simulink library "mblibv1"  (Simulink 6.0)
settings: Solver=ode45  StartTime=0.0  StopTime=10.0  RelTol=1e-3
undefined symbols (not defined in the file or in its folder): gcbh, mech_support
libraries: mblibv1 x10, simulink x5
(part 1 of 2)
settings Model: Creator=batserve  LastModifiedBy=batserve  ExtModeAutoUpdateStatusClock=off
settings Model: ForwardingTableString=|
  | ||__slOldName__||mblibv1/Bodies/Mechanical
  | Environment||__slNewName__||mblibv1/Bodies/Machine
  | Environment||__slOldName__||mblibv1/Utilities/Convert from Pose to
  | Virtual Reality Toolbox||__slNewName__||mblibv1/Utilities/Convert from Rotation Matrix to
  | Virtual Reality Toolbox

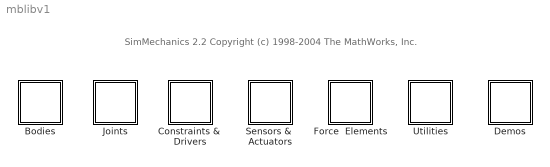
== system mblibv1 ==
  note: SimMechanics 2.2
      | Copyright (c) 1998-2004 The MathWorks, Inc.
  Bodies : Subsystem
      mask Display: image(mech_getIcon('b_lib.bmp', 'Mechanical'))
  Constraints &  Drivers : Subsystem
      mask Display: image(mech_iconLoad('private/constr_lib.bmp'))
  Demos : Subsystem
      settings: OpenFcn=demo('simulink','SimMechanics')
      mask Display: image(mech_getIcon('demo_lib.bmp', 'Mechanical'))
  Force  Elements : Subsystem
      mask Display: image(mech_getIcon('forceelements_lib.bmp', 'Mechanical'))
  Joints : Subsystem
      mask Display: image(mech_getIcon('joint_lib.bmp', 'Mechanical'))
  Sensors &  Actuators : Subsystem
      mask Display: image(mech_getIcon('s_a_lib.bmp', 'Mechanical'))
  Utilities : Subsystem
      mask Display: image(mech_getIcon('conn_lib.bmp', 'Mechanical'))

== system mblibv1/Bodies ==
  Body : PMComponent  LoadFcn=mech_support('LoadFcn',gcbh);  StartFcn=mech_support('StartFcn',gcbh);  StopFcn=mech_support('StopFcn',gcbh);  PhysicalDomain=mechanical  SubClassName=Unknown  LeftPortType=workingframe  RightPortType=workingframe  LConnTagsString=CS1  RConnTagsString=CS2  mask(msb){ClassName=Body, DialogClass=MechanicalBodyBlock, Mass=1, MassUnits=kg, InertiaUnits=kg*m^2, Inertia=eye(3), Shape=Cylinder, ShapeDims=[1 1], ShapeUnits=m, ShapeUse=false, Density=1, DensityUnits=kg/m^3, DensityUse=false, CG=None$CG$[0 0 0]$INERTIAL$INERTIAL$m$[0 0 0]$Euler X-Y-Z$deg$INERTIAL$false, WorkingFrames=Left$CS1$[0 0 0]$CG$CG$m$[0 0 0]$Euler X-Y-Z$deg$INERTIAL$true#Right$CS2$[0 0 0]$CG$CG$m$[0 0 0]$Euler X-Y-Z$deg$INERTIAL$true}
      mask prompts: Mass "MASS_VALUE"; MassUnits "MASS_UNITS"; InertiaUnits "INERTIA_UNITS"; Inertia "INERTIA_VALUE"; Shape "BASE_GEOMETRY"; ShapeDims "GEOMETRY_DIMS"; ShapeUnits "GEOMETRY_UNITS"; ShapeUse "GEOMETRY_USE"; Density "DENSITY_VALUE"; DensityUnits "DENSITY_UNITS"; DensityUse "DENSITY_USE"; CG "CG_FRAME"; WorkingFrames "WORKING_FRAMES"
      mask help: Represents a user-defined rigid body. Body defined by mass m, inertia tensor I, and coordinate origins and axes for center of gravity (CG) and other user-specified Body coordinate systems. This dialog sets Body initial position and orientation, unless Body and/or connected Joints are actuated separately.
      mask init:
      | mech_setIcon private/body.bmp
      settings: CopyFcn=mech_support('CopyFcn',gcbh);  DeleteFcn=mech_support('deleteFcn',gcbh);  UndoDeleteFcn=mech_support('undoDeleteFcn',gcbh);  ModelCloseFcn=mech_support('modelCloseFcn',gcbh);  PreSaveFcn=mech_support('PreSaveFcn');  PostSaveFcn=mech_support('PostSaveFcn');  NameChangeFcn=mech_support('nameChangeFcn',gcbh);  OpenFcn=mech_support('openFcn',gcbh);  CloseFcn=mech_support('CloseFcn',gcbh);
      mask Help: web(mech_help('body'))
      mask Display: image(mech_iconLoad('private/body.bmp'),'center');port_label('LConn',1,'CS1');port_label('RConn',1,'CS2');
  Ground : Subsystem  LoadFcn=mech_support('LoadFcn',gcbh);  StartFcn=mech_support('StartFcn',gcbh);  StopFcn=mech_support('StopFcn',gcbh);  Opaque=on  mask(msb){LeftPortType=env, RightPortType=workingframe, PhysicalDomain=Mechanical, DialogClass=GroundBlock, ClassName=Ground, CoordPosition=[0 0 0], CoordPositionUnits=m, StateVectorMgrId=-1, MachineId=[0 0], ShowEnvPort=off}
      mask help: Grounds one side of a Joint to a fixed location in the World coordinate system.
      mask init:
      | mech_initGround('ground', gcbh, MachineId);
      settings: CopyFcn=mech_support('CopyFcn',gcbh);  DeleteFcn=mech_support('deleteFcn',gcbh);  UndoDeleteFcn=mech_support('undoDeleteFcn',gcbh);  ModelCloseFcn=mech_support('modelCloseFcn',gcbh);  PreSaveFcn=mech_support('PreSaveFcn', gcbh);  PostSaveFcn=mech_support('PostSaveFcn',gcbh);  NameChangeFcn=mech_support('nameChangeFcn',gcbh);  OpenFcn=mech_support('openFcn',gcbh);  CloseFcn=mech_support('CloseFcn',gcbh);
      mask Help: web(mech_help('ground'))
      mask StyleString: edit,edit,edit,edit,edit,edit,popup(km|m|cm|mm|mi|ft|in),edit,edit,checkbox
      mask Display: image(mech_getIcon('ground.bmp', 'Mechanical'),'center','on');
  Machine Environment : Subsystem  Tag=Factory ground  DialogController=MECH.DialogSource  Opaque=on  mask(Mechanical){PortType=env, PhysicalDomain=Mechanical, ClassName=Environment, DialogTemplateClass=MECH.MachineEnvironment, SyncWhenCopied=on, Gravity=[0 -9.81 0], GravityUnits=m/s^2, GravityAsSignal=off, Dimensionality=Auto-detect, AnalysisType=Forward dynamics, LinearAssemblyTolerance=0.001, LinearAssemblyToleranceUnits=m, AngularAssemblyTolerance=0.001, AngularAssemblyToleranceUnits=rad, ConstraintSolverType=Stabilizing, ConstraintRelTolerance=0.0001, ConstraintAbsTolerance=0.0001, UseRobustSingularityHandling=off, StatePerturbationType=Adaptive, PerturbationSize=0.001, VisualizeMachine=on}
      mask help: Defines the mechanical simulation environment for the machine to which the block is connected: gravity, dimensionality, analysis mode, constraint solver type, tolerances, linearization, and visualization.
      mask init:
      | mech_environment_block('MaskInitialization', gcbh);
      settings: CopyFcn=mech_environment_block('CopyFcn', gcbh);
      mask Help: web(mech_help('machineenvironment'))
      mask StyleString: edit,edit,edit,edit,edit,edit,popup(km/s^2|m/s^2|cm/s^2|mm/s^2|mi/s^2|ft/s^2|in/s^2),checkbox,popup(2D Only|3D Only|Auto-detect),popup(Forward dynamics|Inverse dynamics|Kinematics|Trimming),edit,popup(km|m|cm|mm|mi|ft|in),edit,popup(deg|rad),popup(Stabilizing|Tolerancing|Machine precision),edit,edit,checkbox,popup(Adaptive|Fixed),edit,checkbox
      mask Display: disp('Env')

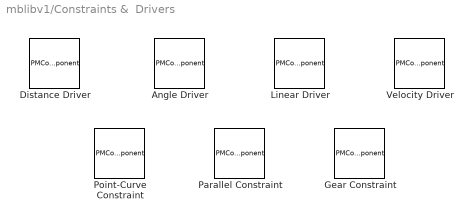
== system mblibv1/Constraints &  Drivers ==
  Angle Driver : PMComponent  LoadFcn=mech_support('LoadFcn',gcbh);  StartFcn=mech_support('StartFcn',gcbh);  StopFcn=mech_support('StopFcn',gcbh);  PhysicalDomain=mechanical  SubClassName=Unknown  LeftPortType=blob  RightPortType=blob  LConnTagsString=__newl0  RConnTagsString=__newr0  mask(AngleDriverConstraint){ClassName=AngleDriver, DialogClass=AngleDriverConstraint, NumSAPorts=0, LeftCsys=WORLD, RightCsys=WORLD, LeftAxis=[1 0 0], RightAxis=[1 0 0]}
      mask help: Drives the angle between base (B) and follower (F) Body axis vectors with a specified Driver Actuator signal, which is added to the initial condition. An unactuated Driver holds the angle in its initial state. Fixed axes define body axis vectors in base and follower coordinate systems. Sensor and actuator ports can be added. Base-follower sequence determines sign of forward motion.
      settings: CopyFcn=mech_support('CopyFcn',gcbh);  DeleteFcn=mech_support('deleteFcn',gcbh);  UndoDeleteFcn=mech_support('undoDeleteFcn',gcbh);  ModelCloseFcn=mech_support('modelCloseFcn',gcbh);  NameChangeFcn=mech_support('nameChangeFcn',gcbh);  OpenFcn=mech_support('openFcn',gcbh);  CloseFcn=mech_support('CloseFcn',gcbh);
      mask Help: web(mech_help('angledriver'))
      mask Display: image(mech_getIcon('ang_drvr.bmp', 'Mechanical'),'center');color('magenta'); port_label('LConn',1,'B'); port_label('RConn',1,'F')
  Distance Driver : PMComponent  LoadFcn=mech_support('LoadFcn',gcbh);  StartFcn=mech_support('StartFcn',gcbh);  StopFcn=mech_support('StopFcn',gcbh);  PhysicalDomain=mechanical  SubClassName=Unknown  LeftPortType=blob  RightPortType=blob  LConnTagsString=__newl0  RConnTagsString=__newr0  mask(DistanceDriverConstraint){ClassName=DistanceDriver, DialogClass=DistanceDriverConstraint, NumSAPorts=0}
      mask help: Drives the distance between origins of the base (B) and follower (F) Body coordinate systems with a specified Driver Actuator signal, which is added to the initial condition. An unactuated Driver holds the distance in its initial state. Distance must remain non-negative at all times. Sensor and actuator ports can be added.
      settings: CopyFcn=mech_support('CopyFcn',gcbh);  DeleteFcn=mech_support('deleteFcn',gcbh);  UndoDeleteFcn=mech_support('undoDeleteFcn',gcbh);  ModelCloseFcn=mech_support('modelCloseFcn',gcbh);  NameChangeFcn=mech_support('nameChangeFcn',gcbh);  OpenFcn=mech_support('openFcn',gcbh);  CloseFcn=mech_support('CloseFcn',gcbh);
      mask Help: web(mech_help('distancedriver'))
      mask Display: image(mech_getIcon('dist_drvr.bmp', 'Mechanical'),'center');color('magenta'); port_label('LConn',1,'B'); port_label('RConn',1,'F')
  Gear Constraint : PMComponent  LoadFcn=mech_support('LoadFcn',gcbh);  StartFcn=mech_support('StartFcn',gcbh);  StopFcn=mech_support('StopFcn',gcbh);  PhysicalDomain=mechanical  SubClassName=Unknown  LeftPortType=blob  RightPortType=blob  LConnTagsString=__newl0  RConnTagsString=__newr0  mask(GearConstraint){ClassName=GearConstraint, DialogClass=GearConstraint, NumSAPorts=0, BaseRadius=1, BaseRadiusUnits=m, FollowerRadius=1, FollowerRadiusUnits=m}
      mask help: Constrains the base (B) and follower (F) Bodies to corotate as meshed gears with pitch circles. The base and follower Bodies must be attached to a third, carrier Body by Revolute or Cylindrical Joints. These joints define the gear rotational axes. Sensor ports can be added. Base-follower sequence determines sign of forward motion.
      settings: CopyFcn=mech_support('CopyFcn',gcbh);  DeleteFcn=mech_support('deleteFcn',gcbh);  UndoDeleteFcn=mech_support('undoDeleteFcn',gcbh);  ModelCloseFcn=mech_support('modelCloseFcn',gcbh);  NameChangeFcn=mech_support('nameChangeFcn',gcbh);  OpenFcn=mech_support('openFcn',gcbh);  CloseFcn=mech_support('CloseFcn',gcbh);
      mask Help: web(mech_help('gearconstraint'))
      mask Display: image(mech_getIcon('gear.bmp', 'Mechanical'),'center');color('magenta'); port_label('LConn',1,'B'); port_label('RConn',1,'F')
  Linear Driver : PMComponent  LoadFcn=mech_support('LoadFcn',gcbh);  StartFcn=mech_support('StartFcn',gcbh);  StopFcn=mech_support('StopFcn',gcbh);  PhysicalDomain=mechanical  SubClassName=Unknown  LeftPortType=blob  RightPortType=blob  LConnTagsString=__newl0  RConnTagsString=__newr0  mask(LinearDriverConstraint){ClassName=LinearDriver, DialogClass=LinearDriverConstraint, NumSAPorts=0, GlobalCoordinate=X}
      mask help: Drives one component [X, Y, or Z] of the relative vector between the origins of the base (B) and follower (F) Body coordinate systems with a Driver Actuator signal, which is added to the initial condition. An unactuated Driver holds the component in its initial state. Vector component measured with respect to the World coordinate system. Follower is the head and base is the tail of relative vector. Sensor and actuator ports can be added. Base-follower sequence determines sign of forward motion, including relative vector component signs.
      settings: CopyFcn=mech_support('CopyFcn',gcbh);  DeleteFcn=mech_support('deleteFcn',gcbh);  UndoDeleteFcn=mech_support('undoDeleteFcn',gcbh);  ModelCloseFcn=mech_support('modelCloseFcn',gcbh);  NameChangeFcn=mech_support('nameChangeFcn',gcbh);  OpenFcn=mech_support('openFcn',gcbh);  CloseFcn=mech_support('CloseFcn',gcbh);
      mask Help: web(mech_help('lineardriver'))
      mask Display: image(mech_getIcon('lin_drvr.bmp', 'Mechanical'),'center');color('magenta'); port_label('LConn',1,'B'); port_label('RConn',1,'F')
  Parallel Constraint : PMComponent  LoadFcn=mech_support('LoadFcn',gcbh);  StartFcn=mech_support('StartFcn',gcbh);  StopFcn=mech_support('StopFcn',gcbh);  PhysicalDomain=mechanical  SubClassName=Unknown  LeftPortType=blob  RightPortType=blob  LConnTagsString=__newl0  RConnTagsString=__newr0  mask(ParallelConstraint){ClassName=ParallelConstraint, DialogClass=ParallelConstraint, NumSAPorts=0, Csys=WORLD, Axis=[1 0 0]}
      mask help: Constrains one Body axis vector defined on both base (B) and follower (F) Bodies to remain parallel. Parallel constraint axis defines initial direction of both Body axis vectors in base and follower Body coordinate systems. Sensor ports can be added. Base-follower sequence determines sign of forward motion.
      settings: CopyFcn=mech_support('CopyFcn',gcbh);  DeleteFcn=mech_support('deleteFcn',gcbh);  UndoDeleteFcn=mech_support('undoDeleteFcn',gcbh);  ModelCloseFcn=mech_support('modelCloseFcn',gcbh);  NameChangeFcn=mech_support('nameChangeFcn',gcbh);  OpenFcn=mech_support('openFcn',gcbh);  CloseFcn=mech_support('CloseFcn',gcbh);
      mask Help: web(mech_help('parallelconstraint'))
      mask Display: image(mech_getIcon('parallel.bmp', 'Mechanical'),'center');color('magenta'); port_label('LConn',1,'B'); port_label('RConn',1,'F')
  Point-Curve Constraint : PMComponent  LoadFcn=mech_support('LoadFcn',gcbh);  StartFcn=mech_support('StartFcn',gcbh);  StopFcn=mech_support('StopFcn',gcbh);  PhysicalDomain=mechanical  SubClassName=Unknown  LeftPortType=blob  RightPortType=blob  LConnTagsString=__newl0  RConnTagsString=__newr0  mask(PointCurveConstraint){ClassName=PointCurve, DialogClass=PointCurveConstraint, Units=m, Xbreaks=[  ], Ybreaks=[  ], Zbreaks=[  ], EndConditions=natural, CanExtrapolate=off, NumSAPorts=0}
      mask help: Constrains the Body coordinate system origin on Body (B) to move along a curve defined in the Body coordinate system on Body (F). The curve is defined as a spline with breakpoints. Sensor ports can be added. Base-follower sequence determines sign of forward motion.
      settings: CopyFcn=mech_support('CopyFcn',gcbh);  DeleteFcn=mech_support('deleteFcn',gcbh);  UndoDeleteFcn=mech_support('undoDeleteFcn',gcbh);  ModelCloseFcn=mech_support('modelCloseFcn',gcbh);  NameChangeFcn=mech_support('nameChangeFcn',gcbh);  OpenFcn=mech_support('openFcn',gcbh);  CloseFcn=mech_support('CloseFcn',gcbh);
      mask Help: web(mech_help('pointcurveconstraint'))
      mask Display: color('magenta');image(mech_getIcon('pt_curve.bmp','Mechanical'),'center');port_label('LConn',1,'B'); port_label('RConn',1,'F')
  Velocity Driver : PMComponent  LoadFcn=mech_support('LoadFcn',gcbh);  StartFcn=mech_support('StartFcn',gcbh);  StopFcn=mech_support('StopFcn',gcbh);  PhysicalDomain=mechanical  SubClassName=Unknown  LeftPortType=blob  RightPortType=blob  LConnTagsString=__newl0  RConnTagsString=__newr0  mask(ConstantVelocityConstraint){ClassName=ConstantVelocity, DialogClass=ConstantVelocityConstraint, NumSAPorts=0, Unit_V=m/s, Unit_Omega=deg/s, Coef_V_Base=[1 0 0], Csys_V_Base=WORLD, Coef_Omega_Base=[1 0 0], Csys_Omega_Base=WORLD, Coef_V_Follower=[1 0 0], Csys_V_Follower=WORLD, Coef_Omega_Follower=[1 0 0], Csys_Omega_Follower=WORLD}
      mask help: Drives a linear combination of projected linear and angular velocities of the base (B) and follower (F) Bodies with a specified Driver Actuator signal, which is added to the initial condition. An unactuated Driver holds the linear combination in its initial state. Sensor and actuator ports can be added. Base-follower sequence determines sign of forward motion.
      settings: CopyFcn=mech_support('CopyFcn',gcbh);  DeleteFcn=mech_support('deleteFcn',gcbh);  UndoDeleteFcn=mech_support('undoDeleteFcn',gcbh);  ModelCloseFcn=mech_support('modelCloseFcn',gcbh);  NameChangeFcn=mech_support('nameChangeFcn',gcbh);  OpenFcn=mech_support('openFcn',gcbh);  CloseFcn=mech_support('CloseFcn',gcbh);
      mask Help: web(mech_help('velocitydriver'))
      mask Display: image(mech_getIcon('con_vel.bmp', 'Mechanical'),'center');color('magenta'); port_label('LConn',1,'B'); port_label('RConn',1,'F')

== system mblibv1/Demos ==

== system mblibv1/Force  Elements ==
  Body Spring & Damper : Subsystem  LoadFcn=mech_support('LoadFcn',gcbh);  StartFcn=mech_support('StartFcn',gcbh);  StopFcn=mech_support('StopFcn',gcbh);  mask(msb){ClassName=BodyForceElement, DialogClass=BodySpringDamper, Spring_k=0, Damper_b=0, Offset_x0=0, PositionUnits=m, VelocityUnits=m/s, ForceUnits=N}
      mask help: Models a damped linear oscillator between two Bodies, equivalent to a translational spring and damper. The force F between the bodies is projected along the axis connecting the Body coordinate systems and is a function of the relative displacement r and velocity v of these Body coordinate systems, given by F = -k*(r-r0) - b*v. The parameters r0, k, and b represent the spring's natural length, the spring constant, and the damper constant, respectively.
      mask init:
      | mech_support('MaskInit', gcbh);
      settings: CopyFcn=mech_support('CopyFcn',gcbh);  DeleteFcn=mech_support('deleteFcn',gcbh);  UndoDeleteFcn=mech_support('undoDeleteFcn',gcbh);  ModelCloseFcn=mech_support('modelCloseFcn',gcbh);  NameChangeFcn=mech_support('nameChangeFcn',gcbh);  OpenFcn=mech_support('openFcn',gcbh);  CloseFcn=mech_support('CloseFcn',gcbh);
      mask Help: web(mech_help('bodyspringdamper'))
      mask Display: image(mech_getIcon('body_springdamper.bmp', 'Mechanical'),'center')
  Joint Spring & Damper : Subsystem  LoadFcn=mech_support('LoadFcn',gcbh);  StartFcn=mech_support('StartFcn',gcbh);  StopFcn=mech_support('StopFcn',gcbh);  mask(msb){ClassName=JointSpringDamper, DialogClass=JointSpringDamper, JFEParameters=P1$false$0$0$0$m$m/s$N$rad$rad/s$N-m#P2$false$0$0$0$m$m/s$N$rad$rad/s$N-m#P3$false$0$0$0$m$m/s$N$rad$rad/s$N-m#R1$false$0$0$0$m$m/s$N$rad$rad/s$N-m#R2$false$0$0$0$m$m/s$N$rad$rad/s$N-m#R3$false$0$0$0$m$m/s$N$rad$rad/s$N-m#S$false$0$0$0$m$m/s$N$rad$rad/s$N-m}
      mask help: Models a damped linear oscillator in a Joint connecting two Bodies, equivalent to a translational spring and damper on prismatic primitives and a torsional spring and damper on revolute primitives. The force or torque F between the bodies is a function of the relative linear or angular displacement x and the linear or angular velocity v of the bodies, given by F = -k*(x-x0) - b*v. The parameters x0, k, and b represent the spring offset, spring constant, and damper constant, respectively. Each prismatic and revolute primitive has a separate spring.
      mask init:
      | mech_support('MaskInit', gcbh);
      settings: CopyFcn=mech_support('CopyFcn',gcbh);  DeleteFcn=mech_support('deleteFcn',gcbh);  UndoDeleteFcn=mech_support('undoDeleteFcn',gcbh);  ModelCloseFcn=mech_support('modelCloseFcn',gcbh);  PreSaveFcn=mech_support('PreSaveFcn');  PostSaveFcn=mech_support('PostSaveFcn');  NameChangeFcn=mech_support('nameChangeFcn',gcbh);  OpenFcn=mech_support('openFcn',gcbh);  CloseFcn=mech_support('CloseFcn',gcbh);
      mask Help: web(mech_help('jointspringdamper'))
      mask Display: image(mech_getIcon('joint_springdamper.bmp', 'Mechanical'),'center')

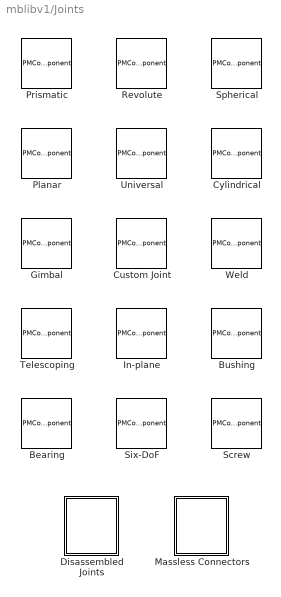
== system mblibv1/Joints ==
  Bearing : PMComponent  LoadFcn=mech_support('LoadFcn',gcbh);  StartFcn=mech_support('StartFcn',gcbh);  StopFcn=mech_support('StopFcn',gcbh);  PhysicalDomain=mechanical  SubClassName=Unknown  LeftPortType=blob  RightPortType=blob  LConnTagsString=__newl0  RConnTagsString=__newr0  mask(msb){NumSAPorts=0, CutJoint=off, MarkAsCut=off, Primitives=revolute_revolute_revolute_prismatic, PrimitiveProps=R1$INERTIAL$[1 0 0]$revolute#R2$INERTIAL$[0 1 0]$revolute#R3$INERTIAL$[0 0 1]$revolute#P1$INERTIAL$[0 0 1]$prismatic, ClassName=BearingJoint, DialogClass=JointBlock}
      mask help: Represents three rotational and one translational degrees of freedom. The follower (F) rotates around three primitive revolute axes (R1, R2, R3) and translates along one primitive prismatic axis P1 with respect to the base (B) Body. Axis P1 must be parallel to axis R3. R1 attached to base. P1 attached to follower. Listed order of primitives is order of motion during simulation. Sensor and actuator ports can be added. Base-follower sequence and axes directions determine sign of forward motion. This joint becomes singular if two revolutes align.
      settings: CopyFcn=mech_support('CopyFcn',gcbh);  DeleteFcn=mech_support('deleteFcn',gcbh);  UndoDeleteFcn=mech_support('undoDeleteFcn',gcbh);  ModelCloseFcn=mech_support('modelCloseFcn',gcbh);  PreSaveFcn=mech_support('PreSaveFcn');  PostSaveFcn=mech_support('PostSaveFcn');  NameChangeFcn=mech_support('nameChangeFcn',gcbh);  OpenFcn=mech_support('openFcn',gcbh);  CloseFcn=mech_support('CloseFcn',gcbh);
      mask Help: web(mech_help('bearing'))
      mask Display: image(mech_getIcon('bearing.bmp', 'Mechanical'),'center');color('red');text(mech_cutAffordance('offset', gcbh) - 2, 0, mech_cutAffordance('text', gcbh),'HorizontalAlignment', 'right','VerticalAlignment', 'bottom');color('magenta');port_label('LConn', 1, 'B');port_label('RConn', 1, 'F');
  Bushing : PMComponent  LoadFcn=mech_support('LoadFcn',gcbh);  StartFcn=mech_support('StartFcn',gcbh);  StopFcn=mech_support('StopFcn',gcbh);  PhysicalDomain=mechanical  SubClassName=Unknown  LeftPortType=blob  RightPortType=blob  LConnTagsString=__newl0  RConnTagsString=__newr0  mask(msb){NumSAPorts=0, CutJoint=off, MarkAsCut=off, Primitives=prismatic_prismatic_prismatic_revolute_revolute_revolute, PrimitiveProps=P1$INERTIAL$[1 0 0]$prismatic#P2$INERTIAL$[0 1 0]$prismatic#P3$INERTIAL$[0 0 1]$prismatic#R1$INERTIAL$[1 0 0]$revolute#R2$INERTIAL$[0 1 0]$revolute#R3$INERTIAL$[0 0 1]$revolute, ClassName=Joint, DialogClass=JointBlock}
      mask help: Represents three rotational and three translational degrees of freedom. The follower (F) translates along three primitive prismatic axes (P1, P2, P3) and rotates around three primitive revolute axes (R1, R2, R3) relative to the base (B) Body. P1 attached to base. R3 attached to follower. Listed order of primitives is order of motion during simulation. Sensor and actuator ports can be added. Base-follower sequence and axes directions determine sign of forward motion. This joint becomes singular if two prismatics or two revolutes align.
      settings: CopyFcn=mech_support('CopyFcn',gcbh);  DeleteFcn=mech_support('deleteFcn',gcbh);  UndoDeleteFcn=mech_support('undoDeleteFcn',gcbh);  ModelCloseFcn=mech_support('modelCloseFcn',gcbh);  PreSaveFcn=mech_support('PreSaveFcn');  PostSaveFcn=mech_support('PostSaveFcn');  NameChangeFcn=mech_support('nameChangeFcn',gcbh);  OpenFcn=mech_support('openFcn',gcbh);  CloseFcn=mech_support('CloseFcn',gcbh);
      mask Help: web(mech_help('bushing'))
      mask Display: image(mech_getIcon('bushing.bmp', 'Mechanical'),'center');color('red');text(mech_cutAffordance('offset', gcbh) - 2, 0, mech_cutAffordance('text', gcbh),'HorizontalAlignment', 'right','VerticalAlignment', 'bottom');color('magenta');port_label('LConn', 1, 'B');port_label('RConn', 1, 'F');
  Custom Joint : PMComponent  LoadFcn=mech_support('LoadFcn',gcbh);  StartFcn=mech_support('StartFcn',gcbh);  StopFcn=mech_support('StopFcn',gcbh);  PhysicalDomain=mechanical  SubClassName=custom_joint  LeftPortType=blob  RightPortType=blob  LConnTagsString=__newl0  RConnTagsString=__newr0  mask(msb){NumSAPorts=0, CutJoint=off, MarkAsCut=off, Primitives=revolute, PrimitiveProps=R1$INERTIAL$[0 0 1]$revolute, ClassName=Joint, DialogClass=JointBlock}
      mask help: Represents general user-defined joint with multiple degrees of freedom. Connects two Bodies with combination of prismatic, revolute, and/or spherical primitives. This Joint limited to maximum of six DoFs: up to three rotational DoFs and up to three translational DoFs. First primitive attached to base (B). Last primitive attached to follower (F). Listed order of primitives is order of motion during simulation. Sensor and actuator ports can be added. Spherical primitive cannot be actuated. Base-follower sequence and axes directions determine sign of forward motion.This joint becomes singular if two prismatics or two revolutes align.
      settings: CopyFcn=mech_support('CopyFcn',gcbh);  DeleteFcn=mech_support('deleteFcn',gcbh);  UndoDeleteFcn=mech_support('undoDeleteFcn',gcbh);  ModelCloseFcn=mech_support('modelCloseFcn',gcbh);  PreSaveFcn=mech_support('PreSaveFcn');  PostSaveFcn=mech_support('PostSaveFcn');  NameChangeFcn=mech_support('nameChangeFcn',gcbh);  OpenFcn=mech_support('openFcn',gcbh);  CloseFcn=mech_support('CloseFcn',gcbh);
      mask Help: web(mech_help('customjoint'))
      mask Display: image(mech_getIcon('comp_joint.bmp', 'Mechanical'),'center');color('red');text(mech_cutAffordance('offset', gcbh) - 2, 0, mech_cutAffordance('text', gcbh),'HorizontalAlignment', 'right','VerticalAlignment', 'bottom');color('magenta');port_label('LConn', 1, 'B');port_label('RConn', 1, 'F');
  Cylindrical : PMComponent  LoadFcn=mech_support('LoadFcn',gcbh);  StartFcn=mech_support('StartFcn',gcbh);  StopFcn=mech_support('StopFcn',gcbh);  PhysicalDomain=mechanical  SubClassName=Unknown  LeftPortType=blob  RightPortType=blob  LConnTagsString=__newl0  RConnTagsString=__newr0  mask(msb){NumSAPorts=0, CutJoint=off, MarkAsCut=off, Primitives=prismatic_revolute, PrimitiveProps=P1$INERTIAL$[1 0 0]$prismatic#R1$INERTIAL$[1 0 0]$revolute, ClassName=CylindricalJoint, DialogClass=JointBlock}
      mask help: Represents one translational and one rotational degrees of freedom. Restricts the follower (F) to move relative to the base (B) Body along and around a common axis P1-R1. Primitive axes P1 and R1 must be aligned. P1 attached to base. R1 attached to follower. Listed order of primitives is order of motion during simulation. Sensor and actuator ports can be added. Base-follower sequence and axis direction determine sign of forward motion.
      settings: CopyFcn=mech_support('CopyFcn',gcbh);  DeleteFcn=mech_support('deleteFcn',gcbh);  UndoDeleteFcn=mech_support('undoDeleteFcn',gcbh);  ModelCloseFcn=mech_support('modelCloseFcn',gcbh);  PreSaveFcn=mech_support('PreSaveFcn');  PostSaveFcn=mech_support('PostSaveFcn');  NameChangeFcn=mech_support('nameChangeFcn',gcbh);  OpenFcn=mech_support('openFcn',gcbh);  CloseFcn=mech_support('CloseFcn',gcbh);
      mask Help: web(mech_help('cylindrical'))
      mask Display: image(mech_getIcon('cylindrical.bmp', 'Mechanical'),'center');color('red');text(mech_cutAffordance('offset', gcbh) - 2, 0, mech_cutAffordance('text', gcbh),'HorizontalAlignment', 'right','VerticalAlignment', 'bottom');color('magenta');port_label('LConn', 1, 'B');port_label('RConn', 1, 'F');
  Disassembled Joints : Subsystem
      mask Display: image(mech_getIcon('joint_lib.bmp', 'Mechanical'))
  Gimbal : PMComponent  LoadFcn=mech_support('LoadFcn',gcbh);  StartFcn=mech_support('StartFcn',gcbh);  StopFcn=mech_support('StopFcn',gcbh);  PhysicalDomain=mechanical  SubClassName=Unknown  LeftPortType=blob  RightPortType=blob  LConnTagsString=__newl0  RConnTagsString=__newr0  mask(msb){NumSAPorts=0, CutJoint=off, MarkAsCut=off, Primitives=revolute_revolute_revolute, PrimitiveProps=R1$INERTIAL$[1 0 0]$revolute#R2$INERTIAL$[0 1 0]$revolute#R3$INERTIAL$[0 0 1]$revolute, ClassName=Joint, DialogClass=JointBlock}
      mask help: Represents three rotational degrees of freedom. The follower (F) rotates with respect to the base (B) Body around three primitive revolute axes (R1, R2, R3). R1 attached to base. R3 attached to follower. Listed order of primitives is order of motion during simulation. Sensor and actuator ports can be added. Base-follower sequence and axes directions determine sign of forward motion. This joint becomes singular if two revolutes align.
      settings: CopyFcn=mech_support('CopyFcn',gcbh);  DeleteFcn=mech_support('deleteFcn',gcbh);  UndoDeleteFcn=mech_support('undoDeleteFcn',gcbh);  ModelCloseFcn=mech_support('modelCloseFcn',gcbh);  PreSaveFcn=mech_support('PreSaveFcn');  PostSaveFcn=mech_support('PostSaveFcn');  NameChangeFcn=mech_support('nameChangeFcn',gcbh);  OpenFcn=mech_support('openFcn',gcbh);  CloseFcn=mech_support('CloseFcn',gcbh);
      mask Help: web(mech_help('gimbal'))
      mask Display: image(mech_getIcon('gimbal.bmp', 'Mechanical'),'center');color('red');text(mech_cutAffordance('offset', gcbh) - 2, 0, mech_cutAffordance('text', gcbh),'HorizontalAlignment', 'right','VerticalAlignment', 'bottom');color('magenta');port_label('LConn', 1, 'B');port_label('RConn', 1, 'F');
  In-plane : PMComponent  LoadFcn=mech_support('LoadFcn',gcbh);  StartFcn=mech_support('StartFcn',gcbh);  StopFcn=mech_support('StopFcn',gcbh);  PhysicalDomain=mechanical  SubClassName=Unknown  LeftPortType=blob  RightPortType=blob  LConnTagsString=__newl0  RConnTagsString=__newr0  mask(msb){NumSAPorts=0, CutJoint=off, MarkAsCut=off, Primitives=prismatic_prismatic, PrimitiveProps=P1$INERTIAL$[1 0 0]$prismatic#P2$INERTIAL$[0 1 0]$prismatic, ClassName=InplaneJoint, DialogClass=JointBlock}
      mask help: Represents two translational degrees of freedom. Restricts the follower (F) to move relative to the base (B) Body in plane defined by span of two primitive prismatic axes (P1, P2). P1 attached to base. P2 attached to follower. Listed order of primitives is order of motion during simulation. Sensor and actuator ports can be added. Base-follower sequence and axes directions determine sign of forward motion. This joint becomes singular if both prismatics align.
      settings: CopyFcn=mech_support('CopyFcn',gcbh);  DeleteFcn=mech_support('deleteFcn',gcbh);  UndoDeleteFcn=mech_support('undoDeleteFcn',gcbh);  ModelCloseFcn=mech_support('modelCloseFcn',gcbh);  PreSaveFcn=mech_support('PreSaveFcn');  PostSaveFcn=mech_support('PostSaveFcn');  NameChangeFcn=mech_support('nameChangeFcn',gcbh);  OpenFcn=mech_support('openFcn',gcbh);  CloseFcn=mech_support('CloseFcn',gcbh);
      mask Help: web(mech_help('inplane'))
      mask Display: image(mech_getIcon('inplane.bmp', 'Mechanical'),'center');color('red');text(mech_cutAffordance('offset', gcbh) - 2, 0, mech_cutAffordance('text', gcbh),'HorizontalAlignment', 'right','VerticalAlignment', 'bottom');color('magenta');port_label('LConn', 1, 'B');port_label('RConn', 1, 'F');
  Massless Connectors : Subsystem
      mask Display: image(mech_getIcon('joint_lib.bmp', 'Mechanical'))
  Planar : PMComponent  LoadFcn=mech_support('LoadFcn',gcbh);  StartFcn=mech_support('StartFcn',gcbh);  StopFcn=mech_support('StopFcn',gcbh);  PhysicalDomain=mechanical  SubClassName=Unknown  LeftPortType=blob  RightPortType=blob  LConnTagsString=__newl0  RConnTagsString=__newr0  mask(msb){NumSAPorts=0, CutJoint=off, MarkAsCut=off, Primitives=prismatic_prismatic_revolute, PrimitiveProps=P1$INERTIAL$[1 0 0]$prismatic#P2$INERTIAL$[0 1 0]$prismatic#R1$INERTIAL$[0 0 1]$revolute, ClassName=PlanarJoint, DialogClass=JointBlock}
      mask help: Represents two translational and one rotational degrees of freedom. Restricts the follower (F) to move relative to the base (B) Body in plane defined by span of two primitive prismatic axes (P1, P2). follower can also rotate about axis R1 = P1 x P2. Axis R1 must be normal to plane. P1 attached to base. R1 attached to follower. Listed order of primitives is order of motion during simulation. Sensor and actuator ports can be added. Base-follower sequence and axes directions determine sign of forward motion. This joint becomes singular if both prismatics align.
      settings: CopyFcn=mech_support('CopyFcn',gcbh);  DeleteFcn=mech_support('deleteFcn',gcbh);  UndoDeleteFcn=mech_support('undoDeleteFcn',gcbh);  ModelCloseFcn=mech_support('modelCloseFcn',gcbh);  PreSaveFcn=mech_support('PreSaveFcn');  PostSaveFcn=mech_support('PostSaveFcn');  NameChangeFcn=mech_support('nameChangeFcn',gcbh);  OpenFcn=mech_support('openFcn',gcbh);  CloseFcn=mech_support('CloseFcn',gcbh);
      mask Help: web(mech_help('planar'))
      mask Display: image(mech_getIcon('planar.bmp', 'Mechanical'),'center');color('red');text(mech_cutAffordance('offset', gcbh) - 2, 0, mech_cutAffordance('text', gcbh),'HorizontalAlignment', 'right','VerticalAlignment', 'bottom');color('magenta');port_label('LConn', 1, 'B');port_label('RConn', 1, 'F');
  Prismatic : PMComponent  LoadFcn=mech_support('LoadFcn',gcbh);  StartFcn=mech_support('StartFcn',gcbh);  StopFcn=mech_support('StopFcn',gcbh);  PhysicalDomain=mechanical  SubClassName=Unknown  LeftPortType=blob  RightPortType=blob  LConnTagsString=__newl0  RConnTagsString=__newr0  mask(msb){NumSAPorts=0, CutJoint=off, MarkAsCut=off, Primitives=prismatic, PrimitiveProps=P1$INERTIAL$[0 0 1]$prismatic, ClassName=Joint, DialogClass=JointBlock}
      mask help: Represents one translational degree of freedom. The follower (F) body translates relative to the base (B) Body along single translational axis connecting Body coordinate origins. Sensor and actuator ports can be added. Base-follower sequence and axis direction determine sign of forward motion.
      settings: CopyFcn=mech_support('CopyFcn',gcbh);  DeleteFcn=mech_support('deleteFcn',gcbh);  UndoDeleteFcn=mech_support('undoDeleteFcn',gcbh);  ModelCloseFcn=mech_support('modelCloseFcn',gcbh);  PreSaveFcn=mech_support('PreSaveFcn');  PostSaveFcn=mech_support('PostSaveFcn');  NameChangeFcn=mech_support('nameChangeFcn',gcbh);  OpenFcn=mech_support('openFcn',gcbh);  CloseFcn=mech_support('CloseFcn',gcbh);
      mask Help: web(mech_help('prismatic'))
      mask Display: image(mech_getIcon('prismatic.bmp', 'Mechanical'),'center');color('red');text(mech_cutAffordance('offset', gcbh) - 2, 0, mech_cutAffordance('text', gcbh),'HorizontalAlignment', 'right','VerticalAlignment', 'bottom');color('magenta');port_label('LConn', 1, 'B');port_label('RConn', 1, 'F');
  Revolute : PMComponent  LoadFcn=mech_support('LoadFcn',gcbh);  StartFcn=mech_support('StartFcn',gcbh);  StopFcn=mech_support('StopFcn',gcbh);  PhysicalDomain=mechanical  SubClassName=Unknown  LeftPortType=blob  RightPortType=blob  LConnTagsString=__newl0  RConnTagsString=__newr0  mask(msb){NumSAPorts=0, CutJoint=off, MarkAsCut=off, Primitives=revolute, PrimitiveProps=R1$INERTIAL$[0 0 1]$revolute, ClassName=Joint, DialogClass=JointBlock}
      mask help: Represents one rotational degree of freedom. The follower (F) Body rotates relative to the base (B) Body about a single rotational axis going through collocated Body coordinate system origins. Sensor and actuator ports can be added. Base-follower sequence and axis direction determine sign of forward motion by the right-hand rule.
      settings: CopyFcn=mech_support('CopyFcn',gcbh);  DeleteFcn=mech_support('deleteFcn',gcbh);  UndoDeleteFcn=mech_support('undoDeleteFcn',gcbh);  ModelCloseFcn=mech_support('modelCloseFcn',gcbh);  PreSaveFcn=mech_support('PreSaveFcn');  PostSaveFcn=mech_support('PostSaveFcn');  NameChangeFcn=mech_support('nameChangeFcn',gcbh);  OpenFcn=mech_support('openFcn',gcbh);  CloseFcn=mech_support('CloseFcn',gcbh);
      mask Help: web(mech_help('revolute'))
      mask Display: image(mech_getIcon('revolute.bmp', 'Mechanical'),'center');color('red');text(mech_cutAffordance('offset', gcbh) - 2, 0, mech_cutAffordance('text', gcbh),'HorizontalAlignment', 'right','VerticalAlignment', 'bottom');color('magenta');port_label('LConn', 1, 'B');port_label('RConn', 1, 'F');
  Screw : PMComponent  LoadFcn=mech_support('LoadFcn',gcbh);  StartFcn=mech_support('StartFcn',gcbh);  StopFcn=mech_support('StopFcn',gcbh);  PhysicalDomain=mechanical  SubClassName=Unknown  LeftPortType=blob  RightPortType=blob  LConnTagsString=__newl0  RConnTagsString=__newr0  mask(msb){NumSAPorts=0, CutJoint=off, MarkAsCut=off, Primitives=revolute, PrimitiveProps=R1$INERTIAL$[1 0 0]$revolute, ClassName=ScrewJoint, DialogClass=ScrewJointBlock, Pitch=1, Units=mm}
      mask help: Represents one translational and one rotational degrees of freedom, with constraint. Restricts the follower (F) to move in helical motion along and around axis R1 relative to the base (B) Body. Translation and rotation constrained to each other by pitch. R1 attached to base and follower. Sensor and actuator ports can be added. Base-follower sequence and axis direction determine sign of forward motion.
      settings: CopyFcn=mech_support('CopyFcn',gcbh);  DeleteFcn=mech_support('deleteFcn',gcbh);  UndoDeleteFcn=mech_support('undoDeleteFcn',gcbh);  ModelCloseFcn=mech_support('modelCloseFcn',gcbh);  PreSaveFcn=mech_support('PreSaveFcn');  PostSaveFcn=mech_support('PostSaveFcn');  NameChangeFcn=mech_support('nameChangeFcn',gcbh);  OpenFcn=mech_support('openFcn',gcbh);  CloseFcn=mech_support('CloseFcn',gcbh);
      mask Help: web(mech_help('screw'))
      mask Display: image(mech_getIcon('screw.bmp', 'Mechanical'),'center');color('red');text(mech_cutAffordance('offset', gcbh) - 2, 0, mech_cutAffordance('text', gcbh),'HorizontalAlignment', 'right','VerticalAlignment', 'bottom');color('magenta');port_label('LConn', 1, 'B');port_label('RConn', 1, 'F');
  Six-DoF : PMComponent  LoadFcn=mech_support('LoadFcn',gcbh);  StartFcn=mech_support('StartFcn',gcbh);  StopFcn=mech_support('StopFcn',gcbh);  PhysicalDomain=mechanical  SubClassName=Unknown  LeftPortType=blob  RightPortType=blob  LConnTagsString=__newl0  RConnTagsString=__newr0  mask(msb){NumSAPorts=0, CutJoint=off, MarkAsCut=off, Primitives=prismatic_prismatic_prismatic_spherical, PrimitiveProps=P1$INERTIAL$[1 0 0]$prismatic#P2$INERTIAL$[0 1 0]$prismatic#P3$INERTIAL$[0 0 1]$prismatic#S$INERTIAL$[0 0 0]$spherical, ClassName=Joint, DialogClass=JointBlock}
      mask help: Represents three translational and three rotational degrees of freedom. Rotational DoFs are in one spherical primitive. Represents most general motion of the follower (F) with respect to the base (B) Body. P1 attached to base. S attached to follower. Listed order of primitives is order of motion during simulation. Sensor and actuator ports can be added. Spherical primitive cannot be actuated. Base-follower sequence and axes directions determine sign of forward motion. This joint becomes singular if two prismatics align.
      settings: CopyFcn=mech_support('CopyFcn',gcbh);  DeleteFcn=mech_support('deleteFcn',gcbh);  UndoDeleteFcn=mech_support('undoDeleteFcn',gcbh);  ModelCloseFcn=mech_support('modelCloseFcn',gcbh);  PreSaveFcn=mech_support('PreSaveFcn');  PostSaveFcn=mech_support('PostSaveFcn');  NameChangeFcn=mech_support('nameChangeFcn',gcbh);  OpenFcn=mech_support('openFcn',gcbh);  CloseFcn=mech_support('CloseFcn',gcbh);
      mask Help: web(mech_help('sixdof'))
      mask Display: image(mech_getIcon('6dof.bmp', 'Mechanical'),'center');color('red');text(mech_cutAffordance('offset', gcbh) - 2, 0, mech_cutAffordance('text', gcbh),'HorizontalAlignment', 'right','VerticalAlignment', 'bottom');color('magenta');port_label('LConn', 1, 'B');port_label('RConn', 1, 'F');
  Spherical : PMComponent  LoadFcn=mech_support('LoadFcn',gcbh);  StartFcn=mech_support('StartFcn',gcbh);  StopFcn=mech_support('StopFcn',gcbh);  PhysicalDomain=mechanical  SubClassName=Unknown  LeftPortType=blob  RightPortType=blob  LConnTagsString=__newl0  RConnTagsString=__newr0  mask(msb){NumSAPorts=0, CutJoint=off, MarkAsCut=off, Primitives=spherical, PrimitiveProps=S$INERTIAL$[0 0 0]$spherical, ClassName=Joint, DialogClass=JointBlock}
      mask help: Represents three rotational degrees of freedom. The follower (F) body pivots freely relative to the base (B) Body at the collocated Body coordinate system origins. Sensor ports can be added. Spherical joint cannot be actuated. Base-follower sequence determines sign of forward motion.
      settings: CopyFcn=mech_support('CopyFcn',gcbh);  DeleteFcn=mech_support('deleteFcn',gcbh);  UndoDeleteFcn=mech_support('undoDeleteFcn',gcbh);  ModelCloseFcn=mech_support('modelCloseFcn',gcbh);  PreSaveFcn=mech_support('PreSaveFcn');  PostSaveFcn=mech_support('PostSaveFcn');  NameChangeFcn=mech_support('nameChangeFcn',gcbh);  OpenFcn=mech_support('openFcn',gcbh);  CloseFcn=mech_support('CloseFcn',gcbh);
      mask Help: web(mech_help('spherical'))
      mask Display: image(mech_getIcon('sphere.bmp', 'Mechanical'),'center');color('red');text(mech_cutAffordance('offset', gcbh) - 2, 0, mech_cutAffordance('text', gcbh),'HorizontalAlignment', 'right','VerticalAlignment', 'bottom');color('magenta');port_label('LConn', 1, 'B');port_label('RConn', 1, 'F');
  Telescoping : PMComponent  LoadFcn=mech_support('LoadFcn',gcbh);  StartFcn=mech_support('StartFcn',gcbh);  StopFcn=mech_support('StopFcn',gcbh);  PhysicalDomain=mechanical  SubClassName=Unknown  LeftPortType=blob  RightPortType=blob  LConnTagsString=__newl0  RConnTagsString=__newr0  mask(msb){NumSAPorts=0, CutJoint=off, MarkAsCut=off, Primitives=spherical_prismatic, PrimitiveProps=S$INERTIAL$[0 0 0]$spherical#P1$INERTIAL$[1 0 0]$prismatic, ClassName=Joint, DialogClass=JointBlock}
      mask help: Represents three rotational and one translational degrees of freedom. Rotational DoFs are in one spherical primitive. The follower (F) pivots freely at collocated Body coordinate system origins and translates along primitive prismatic axis P1 relative to the base (B) Body . S is attached to base. P1 is attached to follower. Listed order of primitives is order of motion during simulation. Sensor and actuator ports can be added. Spherical primitive cannot be actuated. Base-follower sequence and axis direction determine sign of forward motion.
      settings: CopyFcn=mech_support('CopyFcn',gcbh);  DeleteFcn=mech_support('deleteFcn',gcbh);  UndoDeleteFcn=mech_support('undoDeleteFcn',gcbh);  ModelCloseFcn=mech_support('modelCloseFcn',gcbh);  PreSaveFcn=mech_support('PreSaveFcn');  PostSaveFcn=mech_support('PostSaveFcn');  NameChangeFcn=mech_support('nameChangeFcn',gcbh);  OpenFcn=mech_support('openFcn',gcbh);  CloseFcn=mech_support('CloseFcn',gcbh);
      mask Help: web(mech_help('telescoping'))
      mask Display: image(mech_getIcon('telscop.bmp', 'Mechanical'),'center');color('red');text(mech_cutAffordance('offset', gcbh) - 2, 0, mech_cutAffordance('text', gcbh),'HorizontalAlignment', 'right','VerticalAlignment', 'bottom');color('magenta');port_label('LConn', 1, 'B');port_label('RConn', 1, 'F');
  Universal : PMComponent  LoadFcn=mech_support('LoadFcn',gcbh);  StartFcn=mech_support('StartFcn',gcbh);  StopFcn=mech_support('StopFcn',gcbh);  PhysicalDomain=mechanical  SubClassName=Unknown  LeftPortType=blob  RightPortType=blob  LConnTagsString=__newl0  RConnTagsString=__newr0  mask(msb){NumSAPorts=0, CutJoint=off, MarkAsCut=off, Primitives=revolute_revolute, PrimitiveProps=R1$INERTIAL$[0 0 1]$revolute#R2$INERTIAL$[0 1 0]$revolute, ClassName=Joint, DialogClass=JointBlock}
      mask help: Represents two rotational degrees of freedom. The follower (F) rotates with respect to the base (B) Body around two primitive revolute axes (R1, R2). R1 attached to base. R2 attached to follower. Listed order of primitives is order of motion during simulation. Sensor and actuator ports can be added. Base-follower sequence and axes directions determine sign of forward motion. This joint becomes singular if both revolutes align.
      settings: CopyFcn=mech_support('CopyFcn',gcbh);  DeleteFcn=mech_support('deleteFcn',gcbh);  UndoDeleteFcn=mech_support('undoDeleteFcn',gcbh);  ModelCloseFcn=mech_support('modelCloseFcn',gcbh);  PreSaveFcn=mech_support('PreSaveFcn');  PostSaveFcn=mech_support('PostSaveFcn');  NameChangeFcn=mech_support('nameChangeFcn',gcbh);  OpenFcn=mech_support('openFcn',gcbh);  CloseFcn=mech_support('CloseFcn',gcbh);
      mask Help: web(mech_help('universal'))
      mask Display: image(mech_getIcon('universal.bmp', 'Mechanical'),'center');color('red');text(mech_cutAffordance('offset', gcbh) - 2, 0, mech_cutAffordance('text', gcbh),'HorizontalAlignment', 'right','VerticalAlignment', 'bottom');color('magenta');port_label('LConn', 1, 'B');port_label('RConn', 1, 'F');
  Weld : PMComponent  LoadFcn=mech_support('LoadFcn',gcbh);  StartFcn=mech_support('StartFcn',gcbh);  StopFcn=mech_support('StopFcn',gcbh);  PhysicalDomain=mechanical  SubClassName=Unknown  LeftPortType=blob  RightPortType=blob  LConnTagsString=__newl0  RConnTagsString=__newr0  mask(msb){NumSAPorts=0, CutJoint=off, MarkAsCut=off, Primitives=weld, PrimitiveProps=W$INERTIAL$[0 0 0]$weld, ClassName=Joint, DialogClass=JointBlock}
      mask help: Represents zero degrees of freedom. Rigidly connects the base (B) and follower (F) Bodies in initial relative configuration. Sensor ports can be added. Weld joint cannot be actuated.
      settings: CopyFcn=mech_support('CopyFcn',gcbh);  DeleteFcn=mech_support('deleteFcn',gcbh);  UndoDeleteFcn=mech_support('undoDeleteFcn',gcbh);  ModelCloseFcn=mech_support('modelCloseFcn',gcbh);  PreSaveFcn=mech_support('PreSaveFcn');  PostSaveFcn=mech_support('PostSaveFcn');  NameChangeFcn=mech_support('nameChangeFcn',gcbh);  OpenFcn=mech_support('openFcn',gcbh);  CloseFcn=mech_support('CloseFcn',gcbh);
      mask Help: web(mech_help('weld'))
      mask Display: image(mech_getIcon('weld.bmp', 'Mechanical'),'center');color('red');text(mech_cutAffordance('offset', gcbh) - 2, 0, mech_cutAffordance('text', gcbh),'HorizontalAlignment', 'right','VerticalAlignment', 'bottom');color('magenta');port_label('LConn', 1, 'B');port_label('RConn', 1, 'F');
